simulink model "MatFun"  (R2015a)
settings: Solver=ode4  StartTime=0.0  StopTime=15  RelTol=1e-3
settings Model: Creator=HP  LastModifiedBy=HP

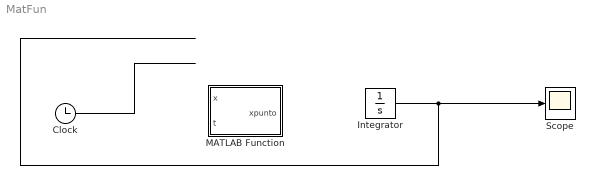
== system MatFun ==
  Clock : Clock
  Integrator : Integrator  InitialCondition=[0 2]
  MATLAB Function : MATLAB Function  TreatAsAtomicUnit=on
  Scope : Scope
  wires:
  Integrator/1 -> Scope/1
  Clock/1 -> ?
  ? -> Integrator/1

== matlab function MatFun/MATLAB Function ==
  data: x input; xpunto output; t input
function xpunto = fcn(x,t)
%#codegen
m=2;
k=1.5;
b=0.2;

A=[0 1;-k/m -b/m];
B=[0;1/m];

u=5;

xpunto = A*x+B*u;
